simulink model "CruiseCon"  (R2020b)
settings: Solver=VariableStepAuto  StartTime=0.0  StopTime=120  RelTol=1e-3
values from neighbouring files (symbols this model uses):
  b = 50    [IntializePara.m]    (also in matlab_Cruise.mat)
  m = 1000    [IntializePara.m]    (also in matlab_Cruise.mat)
settings Model: Creator=BIDITA PAUL  LastModifiedBy=BIDITA PAUL

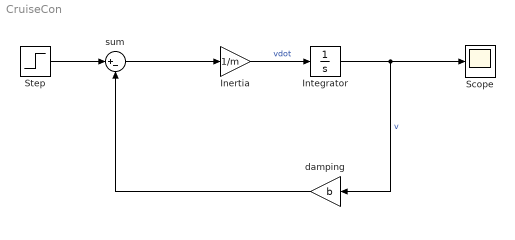
== system CruiseCon ==
  Inertia : Gain  Gain=1/m
  Integrator : Integrator
  Scope : Scope
  Step : Step  After=u  SampleTime=0
  damping : Gain  Gain=b
  sum : Sum  Inputs=|+-
  wires:
  Integrator/1 -> damping/1, Scope/1  "v"
  Inertia/1 -> Integrator/1  "vdot"
  sum/1 -> Inertia/1
  Step/1 -> sum/1
  damping/1 -> sum/2
